simulink library "Lib_HeatXfer_1Dtransconduction2FDE_TMATS_org"  (Simulink 10.0)
settings: Solver=ode45  StartTime=0.0  StopTime=10.0  RelTol=1e-3  EnableMultiTasking=on
Description:
  | Thomas Modules
settings Model: Creator=jwchapm2  LastModifiedBy=bhisma

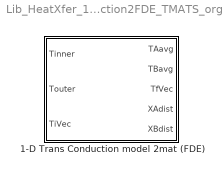
== system Lib_HeatXfer_1Dtransconduction2FDE_TMATS_org ==
  1-D Trans Conduction model 2mat (FDE) : Subsystem  mask(T-MATS: 1-D Trans Cond Model 2mat(FDE) Block){dt_M=4, BlkNm_M=double(gcb), wA_M=4, NodA_M=4, hA_M=1, kA_M=2, rhoA_M=3, cA_M=4, wB_M=4, NodB_M=4, hB_M=1, kB_M=2, rhoB_M=3, cB_M=4}
      mask prompts: dt_M "dt_M - Time Step"; BlkNm_M "BlkNm_M - BlockName"; wA_M "wA_M - Inner Plate Width"; NodA_M "NodA_M - Numer of Nodes"; hA_M "hA_M - convection heat transfer coefficient"; kA_M "kA_M - thermal conductivity"; rhoA_M "rhoA_M - mass density"; cA_M "cA_M - specific heat"; wB_M "wB_M - Outer Plate Width"; NodB_M "NodB_M - Numer of Nodes"; hB_M "hB_M - convection heat transfer coefficient"; kB_M "kB_M - thermal conductivity"; rhoB_M "rhoB_ M - mass density"; cB_M "cB_M - specific heat"
      mask help:
      | This function models the transient conduction of a plate ,consisting of two different materials, A and B coinciding with inner and outer respectively, with fluid on either side via the finite difference method (explicit).
      |
      | Export values are calculated based on a single time step. If additional dynamic behavior is required a simulink memory block may be used to update the temperature initial conditions.
      mask Help: web(which('HeatXfer_TMATS_1DTCond2FDE.html'),'-helpbrowser')

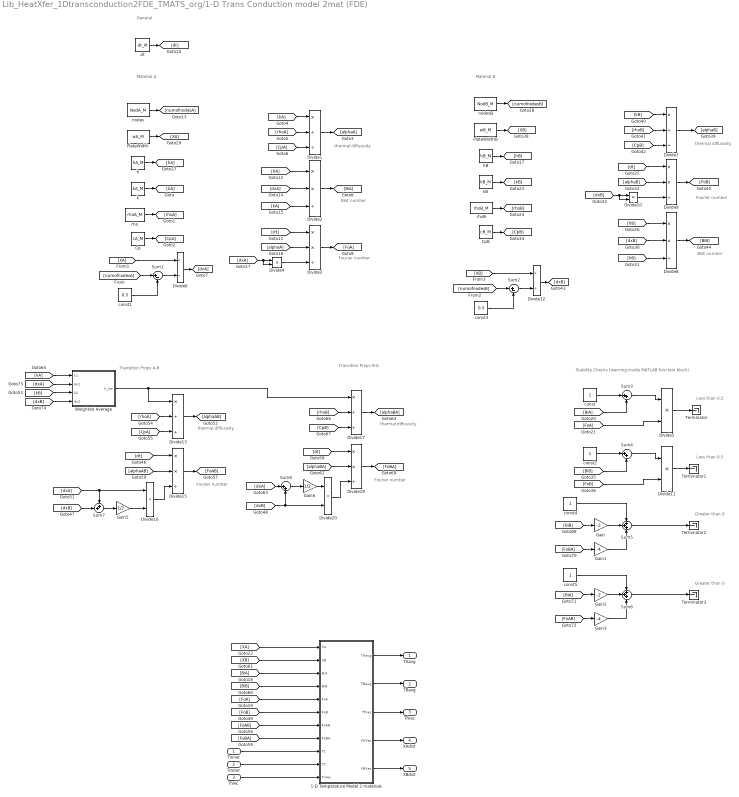
== system Lib_HeatXfer_1Dtransconduction2FDE_TMATS_org/1-D Trans Conduction model 2mat (FDE) ==
  note: Biot number
  note: Fourier number
  note: Fourier number
  note: Fourier number
  note: thermal diffusivity
  note: thermal diffusivity
  note: thermal diffusivity
  note: Greater than 0
  note: Greater than 0
  note: Less than 0.5
  note: Stability Checks (warning inside MATLAB function block)
  note: Transition Props B-A
  note: Transition Props A-B
  note: Material B
  note: Material A
  note: General
  note: Less than 0.5
  note: thermal diffusivity
  note: Fourier number
  note: Biot number
  Tinner : Inport
  Touter : Inport  Port=2
  TiVec : Inport  Port=3
  1-D Temperature Model 2 materials : MATLAB Function  TreatAsAtomicUnit=on
  Cp : Constant  Value=cA_M
  CpB : Constant  Value=cB_M
  Divide{1,7,13,17} (4 alike) : Product  Inputs=*//
  Divide{4..5,10..11,16,20} (6 alike) : Product  Inputs=**
  Divide12 : Product  Inputs=*/
  Divide{2..3,8..9,15,19} (6 alike) : Product  Inputs=**/
  Divide6 : Product  Inputs=*/
  Gain : Gain  Gain=-2
  Gain1 : Gain  Gain=-4
  Gain2 : Gain  Gain=-2
  Gain3 : Gain  Gain=-4
  Gain5 : Gain  Gain=1/2
  Gain6 : Gain  Gain=1/2
  PlateWidth : Constant  Value=wA_M
  PlateWidthB : Constant  Value=wB_M
  Sum1 : Sum  Inputs=|+-
  Sum2 : Sum  Inputs=|+-
  Sum3 : Sum  Inputs=|++
  Sum4 : Sum  Inputs=|++
  Sum5 : Sum  Inputs=+++
  Sum6 : Sum  Inputs=+++
  Sum7 : Sum  Inputs=++|
  Sum8 : Sum  Inputs=|++
  Terminator{,1..3} (4 alike) : Terminator
  Weighted Average : Subsystem
  const{,2,4..5} (4 alike) : Constant
  const1 : Constant  Value=0.5
  const3 : Constant  Value=0.5
  dt : Constant  Value=dt_M
  h : Constant  Value=hA_M
  hB : Constant  Value=hB_M
  k : Constant  Value=kA_M
  kB : Constant  Value=kB_M
  nodes : Constant  Value=NodA_M
  nodesB : Constant  Value=NodB_M
  rho : Constant  Value=rhoA_M
  rhoB : Constant  Value=rhoB_M
  TAavg : Outport
  TBavg : Outport  Port=2
  TfVec : Outport  Port=3
  XAdist : Outport  Port=4
  XBdist : Outport  Port=5
  wires:
  1-D Temperature Model 2 materials/2(TBavg) -> TBavg/1
  Gain3/1 -> Sum6/3
  Gain2/1 -> Sum6/2
  [FoAB] -> Gain3/1
  [BiA] -> Gain2/1
  Sum6/1 -> Terminator3/1
  const5/1 -> Sum6/1
  Gain1/1 -> Sum5/3
  Gain/1 -> Sum5/2
  [FoBA] -> Gain1/1
  [BiB] -> Gain/1
  Sum5/1 -> Terminator2/1
  const4/1 -> Sum5/1
  1-D Temperature Model 2 materials/5(XBVec) -> XBdist/1
  [XB] -> 1-D Temperature Model 2 materials/2(XB)
  [BiB] -> 1-D Temperature Model 2 materials/4(BiB)
  [FoBA] -> 1-D Temperature Model 2 materials/8(FoBA)
  [FoAB] -> 1-D Temperature Model 2 materials/7(FoAB)
  [FoB] -> 1-D Temperature Model 2 materials/6(FoB)
  [dxB] -> Sum8/2, Divide20/2
  [CpB] -> Divide17/3
  [rhoB] -> Divide17/2
  Divide20/1 -> Divide19/3
  Divide17/1 -> [alphaBA]
  Divide19/1 -> [FoBA]
  [alphaBA] -> Divide19/2
  [dt] -> Divide19/1
  [CpA] -> Divide13/3
  [rhoA] -> Divide13/2
  Divide16/1 -> Divide15/3
  Divide13/1 -> [alphaAB]
  Divide15/1 -> [FoAB]
  [dxA] -> Sum7/1, Divide16/1
  [alphaAB] -> Divide15/2
  [dt] -> Divide15/1
  Sum4/1 -> Divide11/1
  [FoB] -> Divide11/2
  [BiB] -> Sum4/2
  Divide11/1 -> Terminator1/1
  [CpB] -> Divide7/3
  [rhoB] -> Divide7/2
  Divide10/1 -> Divide9/3
  const2/1 -> Sum4/1
  [hB] -> Divide8/1
  kB/1 -> [kB]
  rhoB/1 -> [rhoB]
  CpB/1 -> [CpB]
  Divide7/1 -> [alphaB]
  Divide8/1 -> [BiB]
  [kB] -> Divide8/3
  Divide9/1 -> [FoB]
  [kB] -> Divide7/1
  [dxB] -> Divide8/2
  nodesB/1 -> [numofnodesB]
  [dxB] -> Divide10/2, Divide10/1
  [alphaB] -> Divide9/2
  [dt] -> Divide9/1
  hB/1 -> [hB]
  PlateWidthB/1 -> [XB]
  [numofnodesB] -> Sum2/1
  const3/1 -> Sum2/2
  Sum2/1 -> Divide12/2
  [XB] -> Divide12/1
  Divide12/1 -> [dxB]
  Sum3/1 -> Divide5/1
  [XA] -> 1-D Temperature Model 2 materials/1(XA)
  [FoA] -> 1-D Temperature Model 2 materials/5(FoA)
  [FoA] -> Divide5/2
  [BiA] -> Sum3/2
  Divide5/1 -> Terminator/1
  [CpA] -> Divide1/3
  [rhoA] -> Divide1/2
  Divide4/1 -> Divide3/3
  const/1 -> Sum3/1
  [hA] -> Divide2/1
  k/1 -> [kA]
  rho/1 -> [rhoA]
  [BiA] -> 1-D Temperature Model 2 materials/3(BiA)
  Cp/1 -> [CpA]
  Divide1/1 -> [alphaA]
  Divide2/1 -> [BiA]
  [kA] -> Divide2/3
  Divide3/1 -> [FoA]
  [kA] -> Divide1/1
  [dxA] -> Divide2/2
  nodes/1 -> [numofnodesA]
  [dxA] -> Divide4/1, Divide4/2
  dt/1 -> [dt]
  [alphaA] -> Divide3/2
  [dt] -> Divide3/1
  h/1 -> [hA]
  1-D Temperature Model 2 materials/4(XAVec) -> XAdist/1
  1-D Temperature Model 2 materials/3(TfVec) -> TfVec/1
  1-D Temperature Model 2 materials/1(TAavg) -> TAavg/1
  TiVec/1 -> 1-D Temperature Model 2 materials/11(TiVec)
  Tinner/1 -> 1-D Temperature Model 2 materials/9(T1)
  Touter/1 -> 1-D Temperature Model 2 materials/10(T2)
  PlateWidth/1 -> [XA]
  [numofnodesA] -> Sum1/1
  const1/1 -> Sum1/2
  Sum1/1 -> Divide6/2
  [XA] -> Divide6/1
  Divide6/1 -> [dxA]
  Sum7/1 -> Gain5/1
  Gain5/1 -> Divide16/2
  [dxB] -> Sum7/2
  Sum8/1 -> Gain6/1
  [dxA] -> Sum8/1
  Gain6/1 -> Divide20/1
  Weighted Average/1(k_wa) -> Divide13/1, Divide17/1
  [kA] -> Weighted Average/1(k1)
  [kB] -> Weighted Average/3(k2)
  [dxA] -> Weighted Average/2(dx1)
  [dxB] -> Weighted Average/4(dx2)

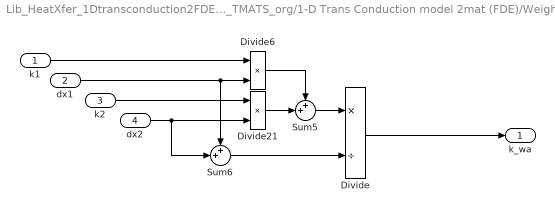
== system Lib_HeatXfer_1Dtransconduction2FDE_TMATS_org/1-D Trans Conduction model 2mat (FDE)/Weighted Average ==
  k1 : Inport
  dx1 : Inport  Port=2
  k2 : Inport  Port=3
  dx2 : Inport  Port=4
  Divide : Product  Inputs=*/
  Divide21 : Product  Inputs=**
  Divide6 : Product  Inputs=**
  Sum5 : Sum  Inputs=++|
  Sum6 : Sum  Inputs=++|
  k_wa : Outport
  wires:
  Sum6/1 -> Divide/2
  k1/1 -> Divide6/1
  Sum5/1 -> Divide/1
  k2/1 -> Divide21/1
  Divide/1 -> k_wa/1
  Divide6/1 -> Sum5/1
  Divide21/1 -> Sum5/2
  dx1/1 -> Divide6/2, Sum6/1
  dx2/1 -> Divide21/2, Sum6/2

== matlab function 1-D Trans Conduction model 2mat (FDE)/1-D Temperature Model 2 materials ==
  data: XA input double; XB input double; BiA input double; TAavg output double; TBavg output double; BiB input double; FoA input double; FoB input double; FoAB input double; FoBA input double; T1 input double; T2 input double; TiVec input double; TfVec output double; XAVec output double; XBVec output double; NodA_M parameter double; NodB_M parameter double; BlkNm_M parameter double
function [TAavg, TBavg,TfVec, XAVec, XBVec] = fcn(XA, XB, BiA, BiB, FoA, FoB, FoAB, FoBA, T1, T2, TiVec, NodA_M, NodB_M, BlkNm_M)
% This function models the heat transfer of a plate (consisting of two
% different materials) with fluid on either side via the finite difference
% method (explicit),
% Per "Fundamentals of Heat and Mass Transfer" 5th edition, Incropera and
% DeWitt, section 5.9
%               |            |              |
%               |            |              |
%               |            |              |
%    Fluid 1    |  Solid A   |    Solid B   |  Fluid 2
%               |            |              |
%               |            |              |
%               |            |              |
%               |            |              |
% Inputs
% T1 - Inner temperature (temperature in contact with A)
% T2 - outer temperature (temperature in contact with B)
% TiVec - initial temperature states
% XA - width of plate A
% XB - width of plate B
% FoA - Fourier number A = alpha * delta_t/ (delta_x)^2
% FoB - Fourier number A = alpha * delta_t/ (delta_x)^2
% FoAB - Fourier number (in material A conduction from material B) = alpha * delta_t/ (delta_x)^2
% FoBA - Fourier number (in material B conduction from material A) = alpha * delta_t/ (delta_x)^2
% BiA - Biot number A = h * delta_x/k
% BiB - Biot number A = h * delta_x/k
% NodA_M - number of nodes for Solid A - 1 (located within the Mask)
% NodB_M - number of nodes for Solid B - 1 (located within the Mask)
% BlkNm_M - name of the block in ACII (located within the Mask)
%
% Outputs
% XAVec - vector of distances from inner -> outer (A)
% XBVec - vector of distances from inner -> outer (B)
% TfVec - output temperature vector
% Tavg - Average Temperature

%Initialize
StatesA = NodA_M;
StatesB = NodB_M;
XAVec = zeros(StatesA,1);
XBVec = zeros(StatesB,1);
NwA = XAVec;
NwB = XBVec;
TfVec = TiVec;
dxA = XA/(StatesA - 1);
dxB = XB/(StatesB - 1);
TAavg = 1;
TBavg = 1;
ii = 1;

% check to determine if all states are stable
if FoA > 0.5
    disp(['Error in block ', BlkNm_M,', FoA > 0.5 , input properties not appropriate for modeling method']);
elseif FoB > 0.5
    disp(['Error in block ', BlkNm_M,', FoB > 0.5 , input properties not appropriate for modeling method']);
elseif FoA*(1+BiA) > 0.5
    disp(['Error in block ', BlkNm_M,', FoA*(1+BiA) > 0.5 , input properties not appropriate for modeling method']);
elseif FoB*(1+BiB) > 0.5
    disp(['Error in block ', BlkNm_M,', FoB*(1+BiB) > 0.5 , input properties not appropriate for modeling method']);
elseif (1 - 2*FoB - 4*FoBA) < 0
    disp(['Error in block ', BlkNm_M,', (1 - 2*FoB - 4*FoBA) < 0 , input properties not appropriate for modeling method']);
elseif (1 - 2*FoA - 4*FoAB) < 0
    disp(['Error in block ', BlkNm_M,', (1 - 2*FoA - 4*FoAB) < 0 , input properties not appropriate for modeling method']);
    
else
    % Calculate each updated node state for material A
    TfVec(1) = 2* FoA * (TiVec(2) + BiA*T1)+ (1 - 2*FoA - 2*BiA*FoA)* TiVec(1);
    XAVec(1) = 0;
    NwA(1) = dxA/2;
    for i = 2: StatesA -1
        TfVec(i) = FoA * (TiVec(i+1) + TiVec(i-1)) + (1 - 2*FoA)*TiVec(i);
        XAVec(i) = XAVec(i-1) + dxA;
        NwA(i) = dxA;
    end
    % transition States A to B
    TfVec(StatesA) = FoA *TiVec(StatesA - 1) + FoAB * TiVec(StatesA + 1)+ (1 - FoA - FoAB)* TiVec(StatesA);
    XAVec(StatesA) = XAVec(StatesA -1) + dxA;
    NwA(StatesA) = dxA;
    % transition States B to A
    TfVec(StatesA + 1) = FoB * TiVec(StatesA + 2) + FoBA * TiVec(StatesA)+ (1 - FoB - FoBA)* TiVec(StatesA + 1);
    XBVec(ii) = dxB/2;
    NwB(ii) = dxB;
    
    % Calculate each updated node state for material B
    for i = (StatesA + 2) : (StatesA + StatesB -1)
        TfVec(i) = FoB * (TiVec(i+1) + TiVec(i-1)) + (1 - 2*FoB)*TiVec(i);
        ii = ii + 1;
        XBVec(ii) = XBVec(ii-1) + dxB;
        NwB(ii) = dxB;
    end
    TfVec(StatesA + StatesB) = 2* FoB * (TiVec(StatesA + StatesB - 1) + BiB*T2)+ (1 - 2*FoB - 2*BiB*FoB)* TiVec(StatesA + StatesB);
    XBVec(StatesB) = XBVec(StatesB -1) + dxB;
    NwB(StatesB) = dxB/2;
    
    TAavg = sum(TfVec(1:StatesA).*NwA)/sum(NwA);
    TBavg = sum(TfVec(StatesA + 1:StatesA + StatesB).*NwB)/sum(NwB);
end
